simulink library "library"  (R2017a)
settings: Solver=VariableStepAuto  StartTime=0.0  StopTime=10.0  RelTol=1e-3
settings Model: Creator=M.Cobb  LastModifiedBy=M.Cobb

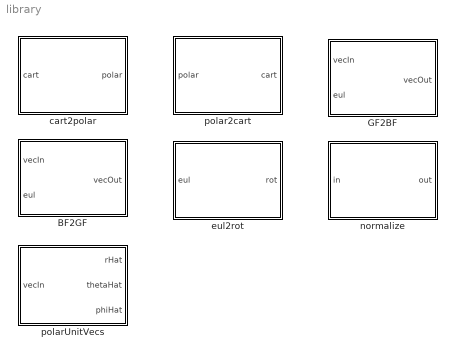
== system library ==
  BF2GF : MATLAB Function  TreatAsAtomicUnit=on
  GF2BF : MATLAB Function  TreatAsAtomicUnit=on
  cart2polar : MATLAB Function  TreatAsAtomicUnit=on
  eul2rot : MATLAB Function  TreatAsAtomicUnit=on
  normalize : MATLAB Function  TreatAsAtomicUnit=on
  polar2cart : MATLAB Function  TreatAsAtomicUnit=on
  polarUnitVecs : MATLAB Function  TreatAsAtomicUnit=on

== matlab function library/GF2BF ==
  data: vecIn input; eul input; vecOut output
function vecOut = GF2BF(vecIn,eul)
% Convert Euler angles to rotation Matrix
yaw   = [cos(eul(1)) -sin(eul(1)) 0; sin(eul(1)) cos(eul(1)) 0;0 0 1];
pitch = [cos(eul(2)) 0 sin(eul(2));0 1 0; -sin(eul(2)) 0 cos(eul(2))];
roll  = [1 0 0;0 cos(eul(3)) -sin(eul(3));0 sin(eul(3)) cos(eul(3))];
vecOut = roll*pitch*yaw*vecIn;
end

== matlab function library/eul2rot ==
  data: eul input; rot output
function rot = eul2rot(eul)
% Convert Euler angles to rotation Matrix
yaw   = [cos(eul(1)) -sin(eul(1)) 0; sin(eul(1)) cos(eul(1)) 0;0 0 1];
pitch = [cos(eul(2)) 0 sin(eul(2));0 1 0; -sin(eul(2)) 0 cos(eul(2))];
roll  = [1 0 0;0 cos(eul(3)) -sin(eul(3));0 sin(eul(3)) cos(eul(3))];
rot = roll*pitch*yaw;
end

== matlab function library/BF2GF ==
  data: vecIn input; eul input; vecOut output
function vecOut = BF2GF(vecIn,eul)
% Convert Euler angles to rotation Matrix
yaw   = [cos(eul(1)) -sin(eul(1)) 0; sin(eul(1)) cos(eul(1)) 0;0 0 1];
pitch = [cos(eul(2)) 0 sin(eul(2));0 1 0; -sin(eul(2)) 0 cos(eul(2))];
roll  = [1 0 0;0 cos(eul(3)) -sin(eul(3));0 sin(eul(3)) cos(eul(3))];
vecOut = (yaw^-1)*(pitch^-1)*(roll^-1)*vecIn;
end

== matlab function library/cart2polar ==
  data: cart input; polar output
function polar = cart2polar(cart)
% convert a ground fixed cartesian vector to polar
% this follows the conventioned outlined here: 
% http://mathworld.wolfram.com/SphericalCoordinates.html
polar = [0;0;0];
% polar(1) = sqrt(sum(cart.^2));
% polar(2) = atan2(cart(2),cart(1));
% polar(3) = (pi/2)-acos(cart(3)/polar(1));
polar(1) = sqrt(sum(vecIn.^2));         %r
polar(2) = atan2(vecIn(2),vecIn(1));    %theta
polar(3) = acos(vecIn(3)/r);            %phi
end

== matlab function library/polar2cart ==
  data: polar input; cart output
function cart = polar2cart(polar)
% convert a ground fixed polar vector to cartesian
% This follows the wolfram convention outlined here:
% http://mathworld.wolfram.com/SphericalCoordinates.html
cart = [0;0;0];
cart(1) = polar(1)*cos(polar(2))*sin(polar(3));
cart(2) = polar(1)*sin(polar(2))*sin(polar(3));
cart(3) = polar(1)*cos(polar(3));
end

== matlab function library/normalize ==
  data: in input; out output
function out = normalize(in)
% normalize a vector
out=in./sqrt(sum(in.^2));
end

== matlab function library/polarUnitVecs ==
  data: vecIn input; rHat output; thetaHat output; phiHat output
function [rHat,thetaHat,phiHat] = polarUnitVecs(vecIn)
% Find ground-frame representation of spherical unit vectors for a given
% cartesian vector.  This follows the wolfram convention outlined here:
% http://mathworld.wolfram.com/SphericalCoordinates.html
r       = sqrt(sum(vecIn.^2));
theta   = atan2(vecIn(2),vecIn(1));
phi     = acos(vecIn(3)/r);

rHat        = [cos(theta)*sin(phi)  sin(theta)*sin(phi) cos(theta)  ];
thetaHat    = [-sin(theta)          cos(theta)          0           ];
phiHat      = [cos(theta)*cos(phi)  sin(theta)*cos(phi) -sin(phi)   ];
end
